simulink model "top_level_sim"  (R2024a)
settings: Solver=FixedStepAuto  StartTime=0.0  StopTime=10.0  FixedStep=0.01  RelTol=1e-3
InitFcn:
  | top_level_sim_init()
model workspace (MAT data in the model file):
  Kp_roll_regulator = 1
values from neighbouring files (symbols this model uses):
  cl03_as_kp = 0    [top_level_sim_init.m]
  cl03_climb_ki = 0    [top_level_sim_init.m]
  cl03_climb_kp = 0    [top_level_sim_init.m]
  cl03_pitch_ki = 0    [top_level_sim_init.m]
  cl03_pitch_kp = 0    [top_level_sim_init.m]
  cl03_roll_kp = 0    [top_level_sim_init.m]
  cl03_yaw_kp = 0    [top_level_sim_init.m]
  S_alphad0_ic_deg = rad2deg(atan2(S_wb0_ic_fps,S_ub0_ic_fps))    [top_level_sim_init.m]
  S_betad0_ic_deg = rad2deg(asin(S_vb0_ic_fps/norm([S_ub0_ic_fps,S_vb0_ic_fps, S_wb0_ic_fps])))    [top_level_sim_init.m]
  S_Ixx_ic_slf2 = 10^6    (= 1000000)    [top_level_sim_init.m]
  S_Ixy_ic_slf2 = 0    [top_level_sim_init.m]
  S_Iyy_ic_slf2 = 10^7    (= 10000000)    [top_level_sim_init.m]
  S_Iyz_ic_slf2 = 0    [top_level_sim_init.m]
  S_Izx_ic_slf2 = 0    [top_level_sim_init.m]
  S_Izz_ic_slf2 = 10^7    (= 10000000)    [top_level_sim_init.m]
  S_mass0_ic_lbs = 300000    [top_level_sim_init.m]
  S_pb0_ic_dps = rad2deg(S_pb0_ic_rps)    [top_level_sim_init.m]
  S_pb0_ic_rps = 0    [top_level_sim_init.m]
  S_phi0_ic_rad = 0    [top_level_sim_init.m]
  S_psi0_ic_rad = 0    [top_level_sim_init.m]
  S_qb0_ic_dps = rad2deg(S_qb0_ic_rps)    [top_level_sim_init.m]
  S_qb0_ic_rps = 0    [top_level_sim_init.m]
  S_rb0_ic_dps = rad2deg(S_rb0_ic_rps)    [top_level_sim_init.m]
  S_rb0_ic_rps = 0    [top_level_sim_init.m]
  S_theta0_ic_rad = 7    [top_level_sim_init.m]
  S_ub0_ic_fps = 5626    [top_level_sim_init.m]
  S_vb0_ic_fps = 0    [top_level_sim_init.m]
  S_wb0_ic_fps = 0    [top_level_sim_init.m]
  S_xi0_ic_ft = 0    [top_level_sim_init.m]
  S_yi0_ic_ft = 0    [top_level_sim_init.m]
  S_zi0_ic_ft = -200    [top_level_sim_init.m]
undefined symbols (not defined in the file or in its folder): CL04_Bmat0, DiscIntNeverNeededParam
libraries: simulink_extras x7, shared6dof x1, aerolibasang x1
settings Model: Creator=chrgutierrez  LastModifiedBy=chrgutierrez
settings DebuggingCC: UnconnectedInputMsg=warning  UnconnectedOutputMsg=warning  UnconnectedLineMsg=warning
settings ModelReferenceCC: EnableRefExpFcnMdlSchedulingChecks=on
settings RTWCC: GPUComputeCapability=3.5  DLArmComputeVersion=19.05

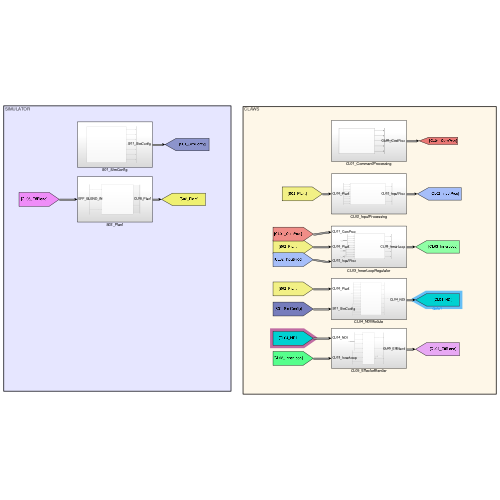
[thumbnail: Simulink's stored preview of the top-level diagram]
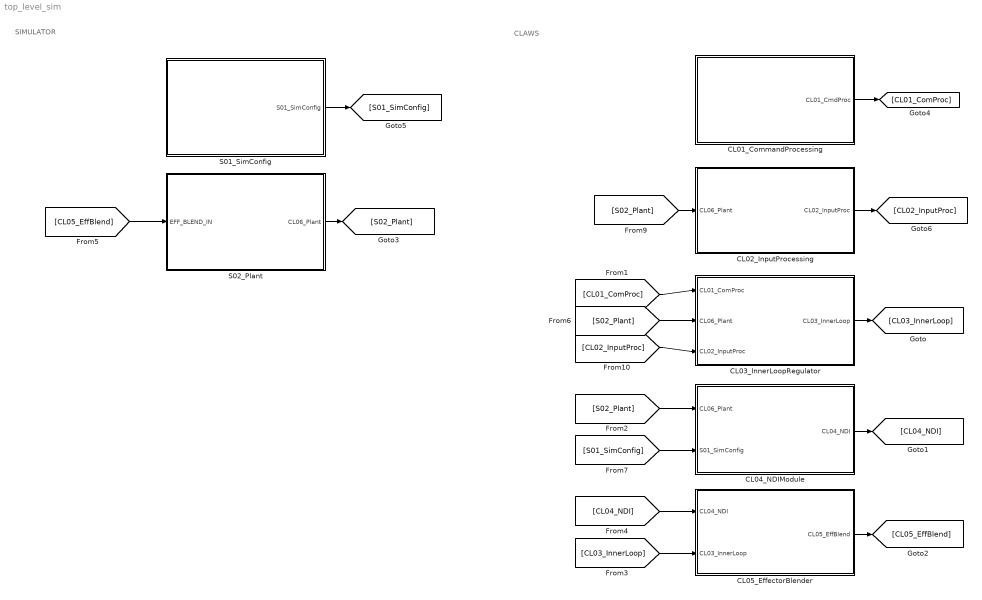
== system top_level_sim ==
  note: CLAWS
  note: SIMULATOR
  CL01_CommandProcessing : Subsystem
  CL02_InputProcessing : Subsystem
  CL03_InnerLoopRegulator : Subsystem
  CL04_NDIModule : Subsystem
  CL05_EffectorBlender : Subsystem
  S01_SimConfig : Subsystem
  S02_Plant : Subsystem
  wires:
  [S02_Plant] -> CL03_InnerLoopRegulator/2(CL06_Plant)
  [CL01_ComProc] -> CL03_InnerLoopRegulator/1(CL01_ComProc)
  CL03_InnerLoopRegulator/1(CL03_InnerLoop) -> [CL03_InnerLoop]
  [CL03_InnerLoop] -> CL05_EffectorBlender/2(CL03_InnerLoop)
  CL04_NDIModule/1(CL04_NDI) -> [CL04_NDI]
  [CL04_NDI] -> CL05_EffectorBlender/1(CL04_NDI)
  CL05_EffectorBlender/1(CL05_EffBlend) -> [CL05_EffBlend]
  [CL05_EffBlend] -> S02_Plant/1(EFF_BLEND_IN)
  [S02_Plant] -> CL04_NDIModule/1(CL06_Plant)
  S01_SimConfig/1(S01_SimConfig) -> [S01_SimConfig]
  [S01_SimConfig] -> CL04_NDIModule/2(S01_SimConfig)
  [S02_Plant] -> CL02_InputProcessing/1(CL06_Plant)
  CL02_InputProcessing/1(CL02_InputProc) -> [CL02_InputProc]
  S02_Plant/1(CL06_Plant) -> [S02_Plant]
  [CL02_InputProc] -> CL03_InnerLoopRegulator/3(CL02_InputProc)
  CL01_CommandProcessing/1(CL01_CmdProc) -> [CL01_ComProc]

== system top_level_sim/CL01_CommandProcessing ==
  Bus Creator : BusCreator  Inputs=5  OutDataTypeStr=Bus: B_CL01_ComProc
      settings: InheritFromInputs=off
  Subsystem : Subsystem
  CL01_CmdProc : Outport
  wires:
  Subsystem/3(rb_cmd_dps) -> Bus Creator/3
  Subsystem/2(qb_cmd_dps) -> Bus Creator/2
  Subsystem/1(pb_cmd_dps) -> Bus Creator/1
  Subsystem/4(as_cmd_fps) -> Bus Creator/4
  Subsystem/5(climb_cmd_fps) -> Bus Creator/5
  Bus Creator/1 -> CL01_CmdProc/1

== system top_level_sim/CL02_InputProcessing ==
  CL06_Plant : Inport
  Bus Creator : BusCreator  Inputs=3  OutDataTypeStr=Bus: B_CL02_InputProcessing
      settings: InheritFromInputs=off
  Bus Selector : BusSelector  OutputSignals=phi_state_rad,theta_state_rad,psi_state_rad,vnorth_state_fps,veast_state_fps,vup_state_fps,ub_state_fps,vb_state_fps,wb_state_fps
  Subsystem : Subsystem
  CL02_InputProc : Outport
  wires:
  CL06_Plant/1 -> Bus Selector/1
  Bus Selector/9 -> Subsystem/9(wb_state_fps)  "<wb_state_fps>"
  Bus Selector/8 -> Subsystem/8(vb_state_fps)  "<vb_state_fps>"
  Bus Selector/7 -> Subsystem/7(ub_state_fps)  "<ub_state_fps>"
  Bus Selector/6 -> Subsystem/6(vup_state_fps)  "<vup_state_fps>"
  Bus Selector/5 -> Subsystem/5(veast_state_fps)  "<veast_state_fps>"
  Bus Selector/4 -> Subsystem/4(vnorth_state_fps)  "<vnorth_state_fps>"
  Bus Selector/3 -> Subsystem/3(psi_state_rad)  "<psi_state_rad>"
  Bus Selector/2 -> Subsystem/2(theta_state_rad)  "<theta_state_rad>"
  Bus Selector/1 -> Subsystem/1(phi_state_rad)  "<phi_state_rad>"
  Subsystem/3(aoa_i_proc_deg) -> Bus Creator/3
  Subsystem/2(aos_i_proc_deg) -> Bus Creator/2
  Subsystem/1(vtot_i_proc_fps) -> Bus Creator/1
  Bus Creator/1 -> CL02_InputProc/1

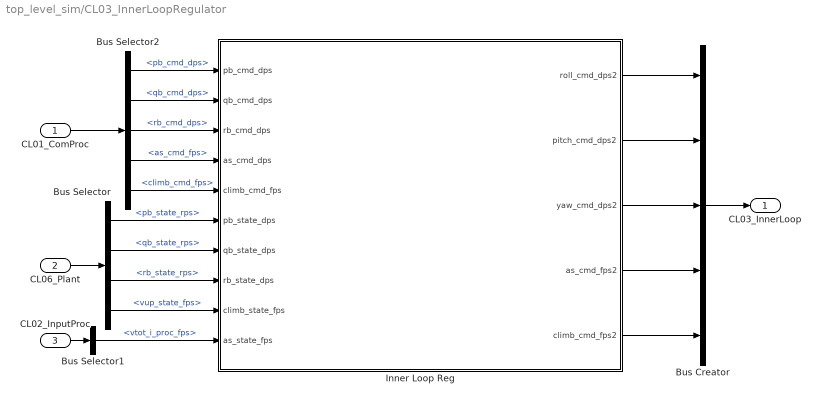
== system top_level_sim/CL03_InnerLoopRegulator ==
  CL01_ComProc : Inport
  CL06_Plant : Inport  Port=2
  CL02_InputProc : Inport  Port=3
  Bus Creator : BusCreator  Inputs=5  OutDataTypeStr=Bus: B_CL03_InnerLoop
      settings: InheritFromInputs=off
  Bus Selector : BusSelector  OutputSignals=pb_state_rps,qb_state_rps,rb_state_rps,vup_state_fps
  Bus Selector1 : BusSelector  OutputSignals=vtot_i_proc_fps
  Bus Selector2 : BusSelector  OutputSignals=pb_cmd_dps,qb_cmd_dps,rb_cmd_dps,as_cmd_fps,climb_cmd_fps
  Inner Loop Reg : Subsystem
  CL03_InnerLoop : Outport
  wires:
  Inner Loop Reg/5(climb_cmd_fps2) -> Bus Creator/5
  Inner Loop Reg/1(roll_cmd_dps2) -> Bus Creator/1
  Inner Loop Reg/4(as_cmd_fps2) -> Bus Creator/4
  Inner Loop Reg/3(yaw_cmd_dps2) -> Bus Creator/3
  Inner Loop Reg/2(pitch_cmd_dps2) -> Bus Creator/2
  Bus Creator/1 -> CL03_InnerLoop/1
  CL06_Plant/1 -> Bus Selector/1
  Bus Selector/1 -> Inner Loop Reg/6(pb_state_dps)  "<pb_state_rps>"
  Bus Selector/2 -> Inner Loop Reg/7(qb_state_dps)  "<qb_state_rps>"
  Bus Selector/3 -> Inner Loop Reg/8(rb_state_dps)  "<rb_state_rps>"
  Bus Selector/4 -> Inner Loop Reg/9(climb_state_fps)  "<vup_state_fps>"
  CL02_InputProc/1 -> Bus Selector1/1
  Bus Selector1/1 -> Inner Loop Reg/10(as_state_fps)  "<vtot_i_proc_fps>"
  CL01_ComProc/1 -> Bus Selector2/1
  Bus Selector2/1 -> Inner Loop Reg/1(pb_cmd_dps)  "<pb_cmd_dps>"
  Bus Selector2/2 -> Inner Loop Reg/2(qb_cmd_dps)  "<qb_cmd_dps>"
  Bus Selector2/3 -> Inner Loop Reg/3(rb_cmd_dps)  "<rb_cmd_dps>"
  Bus Selector2/4 -> Inner Loop Reg/4(as_cmd_dps)  "<as_cmd_fps>"
  Bus Selector2/5 -> Inner Loop Reg/5(climb_cmd_fps)  "<climb_cmd_fps>"

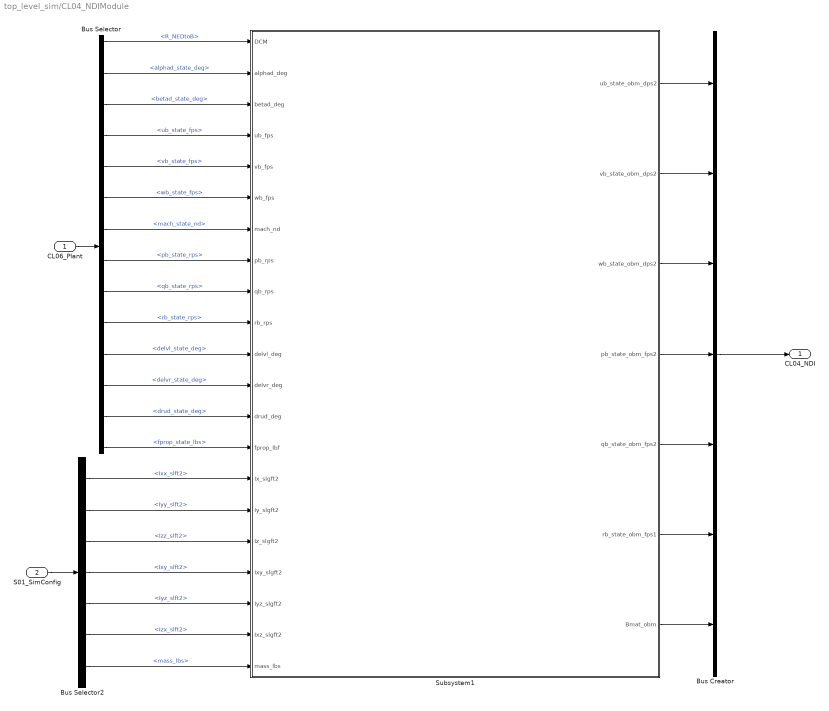
== system top_level_sim/CL04_NDIModule ==
  CL06_Plant : Inport
  S01_SimConfig : Inport  Port=2
  Bus Creator : BusCreator  Inputs=7  OutDataTypeStr=Bus: B_CL04_NDI
      settings: InheritFromInputs=off
  Bus Selector : BusSelector  OutputSignals=R_NEDtoB,alphad_state_deg,betad_state_deg,ub_state_fps,vb_state_fps,wb_state_fps,mach_state_nd,pb_state_rps,qb_state_rps,rb_state_rps,delvl_state_deg,delvr_state_deg,drud_state_deg,fprop_state_lbs
  Bus Selector2 : BusSelector  OutputSignals=Ixx_slft2,Iyy_slft2,Izz_slft2,Ixy_slft2,Iyz_slft2,Izx_slft2,mass_lbs
  Subsystem1 : Subsystem
  CL04_NDI : Outport
  wires:
  CL06_Plant/1 -> Bus Selector/1
  Subsystem1/4(pb_state_obm_fps2) -> Bus Creator/4
  Subsystem1/3(wb_state_obm_dps2) -> Bus Creator/3
  Subsystem1/2(vb_state_obm_dps2) -> Bus Creator/2
  Subsystem1/1(ub_state_obm_dps2) -> Bus Creator/1
  Bus Creator/1 -> CL04_NDI/1
  S01_SimConfig/1 -> Bus Selector2/1
  Bus Selector2/7 -> Subsystem1/21(mass_lbs)  "<mass_lbs>"
  Bus Selector2/1 -> Subsystem1/15(Ix_slgft2)  "<Ixx_slft2>"
  Bus Selector2/2 -> Subsystem1/16(Iy_slgft2)  "<Iyy_slft2>"
  Bus Selector2/3 -> Subsystem1/17(Iz_slgft2)  "<Izz_slft2>"
  Bus Selector2/6 -> Subsystem1/20(Ixz_slgft2)  "<Izx_slft2>"
  Bus Selector2/5 -> Subsystem1/19(Iyz_slgft2)  "<Iyz_slft2>"
  Bus Selector2/4 -> Subsystem1/18(Ixy_slgft2)  "<Ixy_slft2>"
  Bus Selector/2 -> Subsystem1/2(alphad_deg)  "<alphad_state_deg>"
  Bus Selector/3 -> Subsystem1/3(betad_deg)  "<betad_state_deg>"
  Bus Selector/4 -> Subsystem1/4(ub_fps)  "<ub_state_fps>"
  Bus Selector/5 -> Subsystem1/5(vb_fps)  "<vb_state_fps>"
  Bus Selector/6 -> Subsystem1/6(wb_fps)  "<wb_state_fps>"
  Bus Selector/8 -> Subsystem1/8(pb_rps)  "<pb_state_rps>"
  Bus Selector/9 -> Subsystem1/9(qb_rps)  "<qb_state_rps>"
  Bus Selector/10 -> Subsystem1/10(rb_rps)  "<rb_state_rps>"
  Subsystem1/5(qb_state_obm_fps2) -> Bus Creator/5
  Bus Selector/11 -> Subsystem1/11(delvl_deg)  "<delvl_state_deg>"
  Bus Selector/12 -> Subsystem1/12(delvr_deg)  "<delvr_state_deg>"
  Bus Selector/13 -> Subsystem1/13(drud_deg)  "<drud_state_deg>"
  Bus Selector/14 -> Subsystem1/14(fprop_lbf)  "<fprop_state_lbs>"
  Bus Selector/1 -> Subsystem1/1(DCM)  "<R_NEDtoB>"
  Bus Selector/7 -> Subsystem1/7(mach_nd)  "<mach_state_nd>"
  Subsystem1/7(Bmat_obm) -> Bus Creator/7
  Subsystem1/6(rb_state_obm_fps1) -> Bus Creator/6

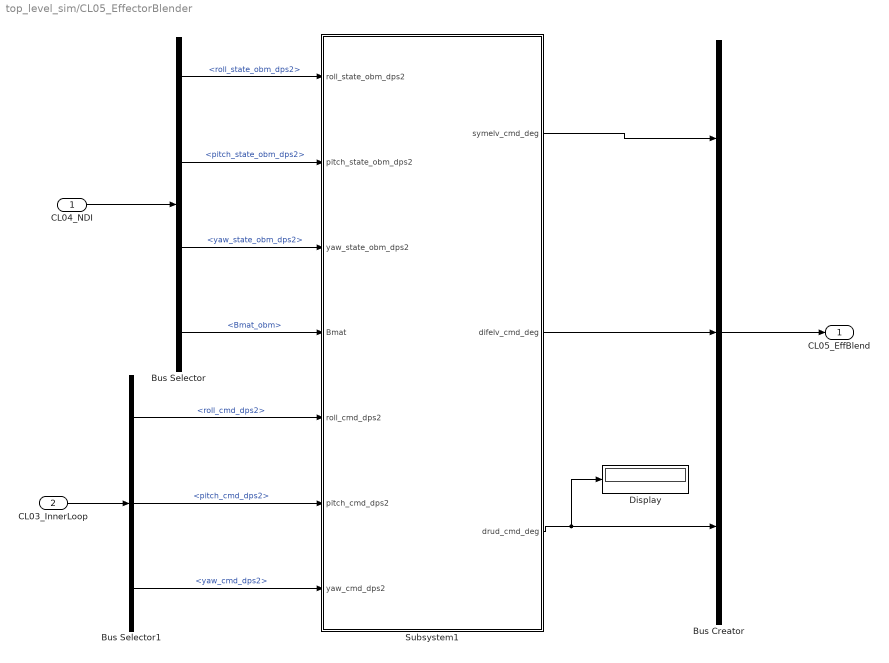
== system top_level_sim/CL05_EffectorBlender ==
  CL04_NDI : Inport
  CL03_InnerLoop : Inport  Port=2
  Bus Creator : BusCreator  Inputs=3  OutDataTypeStr=Bus: B_CL05_EffBlend
      settings: InheritFromInputs=off
  Bus Selector : BusSelector  OutputSignals=roll_state_obm_dps2,pitch_state_obm_dps2,yaw_state_obm_dps2,Bmat_obm
  Bus Selector1 : BusSelector  OutputSignals=roll_cmd_dps2,pitch_cmd_dps2,yaw_cmd_dps2
  Display : Display
  Subsystem1 : Subsystem
  CL05_EffBlend : Outport
  wires:
  CL04_NDI/1 -> Bus Selector/1
  CL03_InnerLoop/1 -> Bus Selector1/1
  Subsystem1/1(symelv_cmd_deg) -> Bus Creator/1
  Subsystem1/2(difelv_cmd_deg) -> Bus Creator/2
  Subsystem1/3(drud_cmd_deg) -> Display/1, Bus Creator/3
  Bus Creator/1 -> CL05_EffBlend/1
  Bus Selector/1 -> Subsystem1/1(roll_state_obm_dps2)  "<roll_state_obm_dps2>"
  Bus Selector/2 -> Subsystem1/2(pitch_state_obm_dps2)  "<pitch_state_obm_dps2>"
  Bus Selector/3 -> Subsystem1/3(yaw_state_obm_dps2)  "<yaw_state_obm_dps2>"
  Bus Selector/4 -> Subsystem1/4(Bmat)  "<Bmat_obm>"
  Bus Selector1/3 -> Subsystem1/7(yaw_cmd_dps2)  "<yaw_cmd_dps2>"
  Bus Selector1/2 -> Subsystem1/6(pitch_cmd_dps2)  "<pitch_cmd_dps2>"
  Bus Selector1/1 -> Subsystem1/5(roll_cmd_dps2)  "<roll_cmd_dps2>"

== system top_level_sim/S01_SimConfig ==
  Bus Creator : BusCreator  Inputs=7  OutDataTypeStr=Bus: B_S01_SimConfig
      settings: InheritFromInputs=off
  Subsystem : Subsystem
  S01_SimConfig : Outport
  wires:
  Bus Creator/1 -> S01_SimConfig/1
  Subsystem/1(mass_lbs) -> Bus Creator/1
  Subsystem/2(Ixx_slft2) -> Bus Creator/2
  Subsystem/3(Iyy_slft2) -> Bus Creator/3
  Subsystem/4(Izz_slft2) -> Bus Creator/4
  Subsystem/5(Ixy_slft2) -> Bus Creator/5
  Subsystem/6(Iyz_slft2) -> Bus Creator/6
  Subsystem/7(Izx_slft2) -> Bus Creator/7

== system top_level_sim/S02_Plant ==
  EFF_BLEND_IN : Inport
  Bus Creator : BusCreator  Inputs=29  OutDataTypeStr=Bus: B_S02_Plant
      settings: InheritFromInputs=off
  Bus Selector : BusSelector  OutputSignals=symelv_cmd_deg,difelv_cmd_deg,drud_cmd_deg
  Subsystem : Subsystem
  CL06_Plant : Outport
  wires:
  Bus Creator/1 -> CL06_Plant/1
  EFF_BLEND_IN/1 -> Bus Selector/1
  Subsystem/1(alphad_deg1) -> Bus Creator/1
  Subsystem/2(betad_deg1) -> Bus Creator/2
  Subsystem/3(delvl_state_deg) -> Bus Creator/3
  Subsystem/4(delvr_state_deg) -> Bus Creator/4
  Subsystem/5(drud_state_deg) -> Bus Creator/5
  Subsystem/6(fprop_state_lbf) -> Bus Creator/6
  Subsystem/7(vnorth_state_fps) -> Bus Creator/7
  Subsystem/8(veast_state_fps) -> Bus Creator/8
  Subsystem/9(vup_state_fps) -> Bus Creator/9
  Subsystem/10(xnorth_state_ft) -> Bus Creator/10
  Subsystem/11(xeast_state_ft) -> Bus Creator/11
  Subsystem/12(xup_state_ft) -> Bus Creator/12
  Subsystem/13(phi_state_rad) -> Bus Creator/13
  Subsystem/14(theta_state_rad) -> Bus Creator/14
  Subsystem/15(psi_state_rad) -> Bus Creator/15
  Subsystem/16(R_NEDtoB) -> Bus Creator/16
  Subsystem/17(ub_state_fps) -> Bus Creator/17
  Subsystem/18(vb_state_fps) -> Bus Creator/18
  Subsystem/19(wb_state_fps) -> Bus Creator/19
  Subsystem/20(pb_state_rps) -> Bus Creator/20
  Subsystem/21(qb_state_rps) -> Bus Creator/21
  Subsystem/22(rb_state_rps) -> Bus Creator/22
  Subsystem/23(pbdot_state_rps2) -> Bus Creator/23
  Subsystem/24(qbdot_state_rps2) -> Bus Creator/24
  Subsystem/25(rbdot_state_rps2) -> Bus Creator/25
  Subsystem/26(axb_state_fps2) -> Bus Creator/26
  Subsystem/27(ayb_state_fps2) -> Bus Creator/27
  Subsystem/28(azb_state_fps2) -> Bus Creator/28
  Bus Selector/2 -> Subsystem/2(difelv_cmd_deg)  "<difelv_cmd_deg>"
  Bus Selector/1 -> Subsystem/1(symelv_cmd_deg)  "<symelv_cmd_deg>"
  Bus Selector/3 -> Subsystem/3(drud_deg)  "<drud_cmd_deg>"
  Subsystem/29(mach_state_nd) -> Bus Creator/29

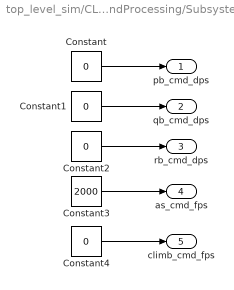
== system top_level_sim/CL01_CommandProcessing/Subsystem ==
  Constant{,1..2,4} (4 alike) : Constant  Value=0
  Constant3 : Constant  Value=2000
  pb_cmd_dps : Outport
  qb_cmd_dps : Outport  Port=2
  rb_cmd_dps : Outport  Port=3
  as_cmd_fps : Outport  Port=4
  climb_cmd_fps : Outport  Port=5
  wires:
  Constant/1 -> pb_cmd_dps/1
  Constant1/1 -> qb_cmd_dps/1
  Constant2/1 -> rb_cmd_dps/1
  Constant3/1 -> as_cmd_fps/1
  Constant4/1 -> climb_cmd_fps/1

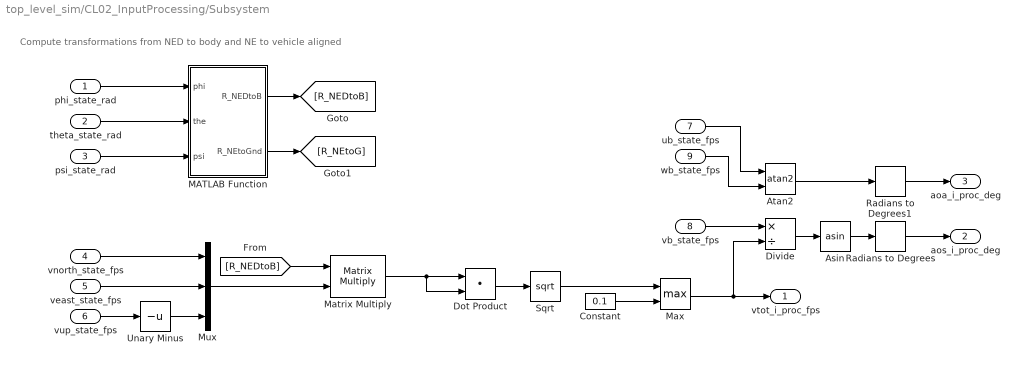
== system top_level_sim/CL02_InputProcessing/Subsystem ==
  note: Compute transformations from NED to body and NE to vehicle aligned
  phi_state_rad : Inport
  theta_state_rad : Inport  Port=2
  psi_state_rad : Inport  Port=3
  vnorth_state_fps : Inport  Port=4
  veast_state_fps : Inport  Port=5
  vup_state_fps : Inport  Port=6
  ub_state_fps : Inport  Port=7
  vb_state_fps : Inport  Port=8
  wb_state_fps : Inport  Port=9
  Asin : Trigonometry  Operator=asin
  Atan2 : Trigonometry  Operator=atan2
  Constant : Constant  Value=0.1
  Divide : Product  Inputs=*/
  Dot Product : DotProduct  OutDataTypeStr=Inherit: Inherit via internal rule
  MATLAB Function : MATLAB Function  TreatAsAtomicUnit=on
  Matrix Multiply : Product  Multiplication=Matrix(*)
  Max : MinMax  Function=max  Inputs=2
  Mux : Mux  Inputs=3
  Radians to Degrees : simulink_extras/Transformations/Radians to Degrees
  Radians to Degrees1 : simulink_extras/Transformations/Radians to Degrees
  Sqrt : Sqrt
  Unary Minus : UnaryMinus
  vtot_i_proc_fps : Outport
  aos_i_proc_deg : Outport  Port=2
  aoa_i_proc_deg : Outport  Port=3
  wires:
  psi_state_rad/1 -> MATLAB Function/3(psi)
  theta_state_rad/1 -> MATLAB Function/2(the)
  phi_state_rad/1 -> MATLAB Function/1(phi)
  MATLAB Function/2(R_NEtoGnd) -> [R_NEtoG]
  MATLAB Function/1(R_NEDtoB) -> [R_NEDtoB]
  vup_state_fps/1 -> Unary Minus/1
  veast_state_fps/1 -> Mux/2
  vnorth_state_fps/1 -> Mux/1
  Unary Minus/1 -> Mux/3
  Mux/1 -> Matrix Multiply/2
  [R_NEDtoB] -> Matrix Multiply/1
  Matrix Multiply/1 -> Dot Product/1, Dot Product/2
  Dot Product/1 -> Sqrt/1
  Sqrt/1 -> Max/1
  Constant/1 -> Max/2
  Max/1 -> vtot_i_proc_fps/1, Divide/2
  vb_state_fps/1 -> Divide/1
  Divide/1 -> Asin/1
  Asin/1 -> Radians to Degrees/1
  Radians to Degrees/1 -> aos_i_proc_deg/1
  wb_state_fps/1 -> Atan2/2
  ub_state_fps/1 -> Atan2/1
  Atan2/1 -> Radians to Degrees1/1
  Radians to Degrees1/1 -> aoa_i_proc_deg/1

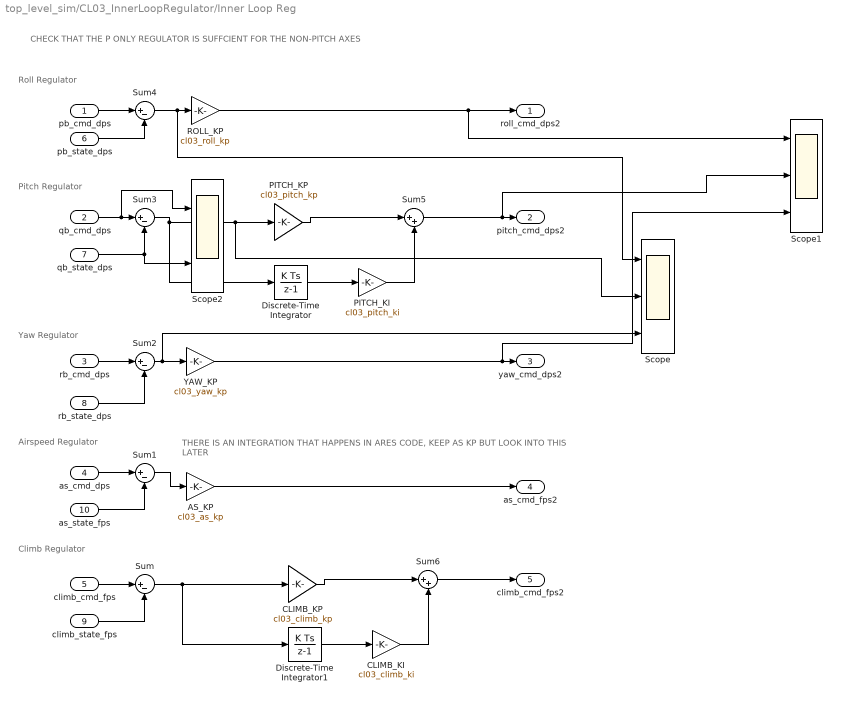
== system top_level_sim/CL03_InnerLoopRegulator/Inner Loop Reg ==
  note: THERE IS AN INTEGRATION THAT HAPPENS IN ARES CODE, KEEP AS KP BUT LOOK INTO THIS LATER
  note: CHECK THAT THE P ONLY REGULATOR IS SUFFCIENT FOR THE NON-PITCH AXES
  note: Roll Regulator
  note: Pitch Regulator
  note: Yaw Regulator
  note: Airspeed Regulator
  note: Climb Regulator
  pb_cmd_dps : Inport
  qb_cmd_dps : Inport  Port=2
  rb_cmd_dps : Inport  Port=3
  as_cmd_dps : Inport  Port=4
  climb_cmd_fps : Inport  Port=5
  pb_state_dps : Inport  Port=6
  qb_state_dps : Inport  Port=7
  rb_state_dps : Inport  Port=8
  climb_state_fps : Inport  Port=9
  as_state_fps : Inport  Port=10
  AS_KP : Gain  Gain=cl03_as_kp
  CLIMB_KI : Gain  Gain=cl03_climb_ki
  CLIMB_KP : Gain  Gain=cl03_climb_kp
  Discrete-Time Integrator : DiscreteIntegrator  SampleTime=-1  ICPrevOutput=DiscIntNeverNeededParam  ICPrevScaledInput=DiscIntNeverNeededParam
  Discrete-Time Integrator1 : DiscreteIntegrator  SampleTime=-1  ICPrevOutput=DiscIntNeverNeededParam  ICPrevScaledInput=DiscIntNeverNeededParam
  PITCH_KI : Gain  Gain=cl03_pitch_ki
  PITCH_KP : Gain  Gain=cl03_pitch_kp
  ROLL_KP : Gain  Gain=cl03_roll_kp
  Scope : Scope  NumInputPorts=3
  Scope1 : Scope  NumInputPorts=3
  Scope2 : Scope  NumInputPorts=2
  Sum{,1..4} (5 alike) : Sum  Inputs=|+-
  Sum5 : Sum  Inputs=|++
  Sum6 : Sum  Inputs=|++
  YAW_KP : Gain  Gain=cl03_yaw_kp
  roll_cmd_dps2 : Outport
  pitch_cmd_dps2 : Outport  Port=2
  yaw_cmd_dps2 : Outport  Port=3
  as_cmd_fps2 : Outport  Port=4
  climb_cmd_fps2 : Outport  Port=5
  wires:
  climb_cmd_fps/1 -> Sum/1
  climb_state_fps/1 -> Sum/2
  as_cmd_dps/1 -> Sum1/1
  as_state_fps/1 -> Sum1/2
  rb_cmd_dps/1 -> Sum2/1
  rb_state_dps/1 -> Sum2/2
  qb_cmd_dps/1 -> Scope2/1, Sum3/1
  qb_state_dps/1 -> Scope2/2, Sum3/2
  pb_cmd_dps/1 -> Sum4/1
  pb_state_dps/1 -> Sum4/2
  Sum4/1 -> Scope/1, ROLL_KP/1
  ROLL_KP/1 -> Scope1/1, roll_cmd_dps2/1
  Sum2/1 -> Scope/3, YAW_KP/1
  YAW_KP/1 -> Scope1/3, yaw_cmd_dps2/1
  Sum1/1 -> AS_KP/1
  AS_KP/1 -> as_cmd_fps2/1
  Discrete-Time Integrator/1 -> PITCH_KI/1
  PITCH_KI/1 -> Sum5/2
  PITCH_KP/1 -> Sum5/1
  Sum5/1 -> Scope1/2, pitch_cmd_dps2/1
  Sum3/1 -> Scope/2, PITCH_KP/1, Discrete-Time Integrator/1
  Sum/1 -> CLIMB_KP/1, Discrete-Time Integrator1/1
  Sum6/1 -> climb_cmd_fps2/1
  CLIMB_KI/1 -> Sum6/2
  Discrete-Time Integrator1/1 -> CLIMB_KI/1
  CLIMB_KP/1 -> Sum6/1

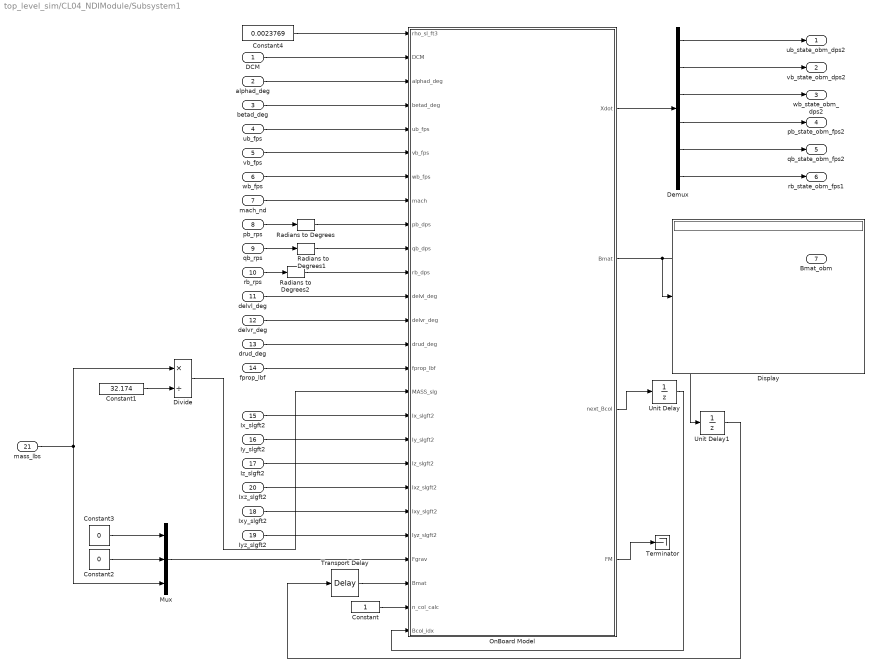
== system top_level_sim/CL04_NDIModule/Subsystem1 ==
  DCM : Inport
  alphad_deg : Inport  Port=2
  betad_deg : Inport  Port=3
  ub_fps : Inport  Port=4
  vb_fps : Inport  Port=5
  wb_fps : Inport  Port=6
  mach_nd : Inport  Port=7
  pb_rps : Inport  Port=8
  qb_rps : Inport  Port=9
  rb_rps : Inport  Port=10
  delvl_deg : Inport  Port=11
  delvr_deg : Inport  Port=12
  drud_deg : Inport  Port=13
  fprop_lbf : Inport  Port=14
  Ix_slgft2 : Inport  Port=15
  Iy_slgft2 : Inport  Port=16
  Iz_slgft2 : Inport  Port=17
  Ixy_slgft2 : Inport  Port=18
  Iyz_slgft2 : Inport  Port=19
  Ixz_slgft2 : Inport  Port=20
  mass_lbs : Inport  Port=21
  Constant : Constant
  Constant1 : Constant  Value=32.174
  Constant2 : Constant  Value=0
  Constant3 : Constant  Value=0
  Constant4 : Constant  Value=0.0023769
  Demux : Demux  Outputs=6
  Display : Display
  Divide : Product  Inputs=*/
  Mux : Mux  Inputs=3
  OnBoard Model : MATLAB Function  TreatAsAtomicUnit=on
  Radians to Degrees : simulink_extras/Transformations/Radians to Degrees
  Radians to Degrees1 : simulink_extras/Transformations/Radians to Degrees
  Radians to Degrees2 : simulink_extras/Transformations/Radians to Degrees
  Terminator : Terminator
  Transport Delay : TransportDelay  DelayTime=3  InitialOutput=CL04_Bmat0
  Unit Delay : UnitDelay  SampleTime=-1  HasFrameUpgradeWarning=on
  Unit Delay1 : UnitDelay  SampleTime=-1  HasFrameUpgradeWarning=on
  ub_state_obm_dps2 : Outport
  vb_state_obm_dps2 : Outport  Port=2
  wb_state_obm_dps2 : Outport  Port=3
  pb_state_obm_fps2 : Outport  Port=4
  qb_state_obm_fps2 : Outport  Port=5
  rb_state_obm_fps1 : Outport  Port=6
  Bmat_obm : Outport  Port=7
  wires:
  OnBoard Model/3(next_Bcol) -> Unit Delay/1
  OnBoard Model/2(Bmat) -> Display/1, Unit Delay1/1, Bmat_obm/1
  OnBoard Model/4(FM) -> Terminator/1
  OnBoard Model/1(Xdot) -> Demux/1
  Unit Delay/1 -> OnBoard Model/26(Bcol_idx)
  Demux/3 -> wb_state_obm_dps2/1
  Demux/1 -> ub_state_obm_dps2/1
  Demux/2 -> vb_state_obm_dps2/1
  Demux/4 -> pb_state_obm_fps2/1
  Demux/5 -> qb_state_obm_fps2/1
  Unit Delay1/1 -> Transport Delay/1
  Constant/1 -> OnBoard Model/25(n_col_calc)
  wb_fps/1 -> OnBoard Model/7(wb_fps)
  vb_fps/1 -> OnBoard Model/6(vb_fps)
  ub_fps/1 -> OnBoard Model/5(ub_fps)
  Ix_slgft2/1 -> OnBoard Model/17(Ix_slgft2)
  Iy_slgft2/1 -> OnBoard Model/18(Iy_slgft2)
  Iz_slgft2/1 -> OnBoard Model/19(Iz_slgft2)
  Ixz_slgft2/1 -> OnBoard Model/20(Ixz_slgft2)
  Ixy_slgft2/1 -> OnBoard Model/21(Ixy_slgft2)
  Iyz_slgft2/1 -> OnBoard Model/22(Iyz_slgft2)
  delvl_deg/1 -> OnBoard Model/12(delvl_deg)
  drud_deg/1 -> OnBoard Model/14(drud_deg)
  delvr_deg/1 -> OnBoard Model/13(delvr_deg)
  pb_rps/1 -> Radians to Degrees/1
  Radians to Degrees/1 -> OnBoard Model/9(pb_dps)
  qb_rps/1 -> Radians to Degrees1/1
  Radians to Degrees1/1 -> OnBoard Model/10(qb_dps)
  rb_rps/1 -> Radians to Degrees2/1
  Radians to Degrees2/1 -> OnBoard Model/11(rb_dps)
  alphad_deg/1 -> OnBoard Model/3(alphad_deg)
  betad_deg/1 -> OnBoard Model/4(betad_deg)
  Constant1/1 -> Divide/2
  mass_lbs/1 -> Divide/1, Mux/3
  Divide/1 -> OnBoard Model/16(MASS_slg)
  fprop_lbf/1 -> OnBoard Model/15(fprop_lbf)
  Constant3/1 -> Mux/1
  Constant2/1 -> Mux/2
  Mux/1 -> OnBoard Model/23(Fgrav)
  DCM/1 -> OnBoard Model/2(DCM)
  Constant4/1 -> OnBoard Model/1(rho_sl_ft3)
  mach_nd/1 -> OnBoard Model/8(mach)
  Demux/6 -> rb_state_obm_fps1/1
  Transport Delay/1 -> OnBoard Model/24("Bmat ")

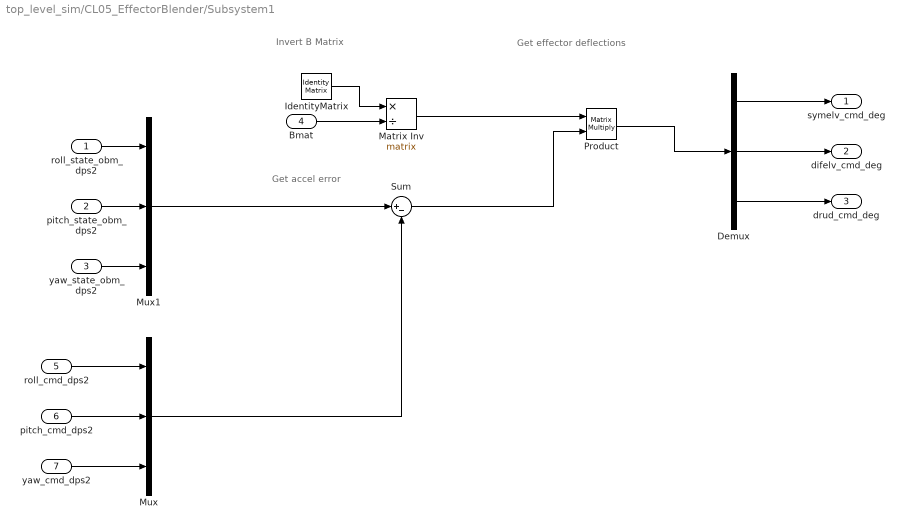
== system top_level_sim/CL05_EffectorBlender/Subsystem1 ==
  note: Get accel error
  note: Invert B Matrix
  note: Get effector deflections
  roll_state_obm_dps2 : Inport
  pitch_state_obm_dps2 : Inport  Port=2
  yaw_state_obm_dps2 : Inport  Port=3
  Bmat : Inport  Port=4
  roll_cmd_dps2 : Inport  Port=5
  pitch_cmd_dps2 : Inport  Port=6
  yaw_cmd_dps2 : Inport  Port=7
  Demux : Demux  Outputs=3
  IdentityMatrix : IdentityMatrix  OutputDimensions=3
  Matrix Inv : Product  Inputs=*/  Multiplication=Matrix(*)
  Mux : Mux  Inputs=3
  Mux1 : Mux  Inputs=3
  Product : Product  Multiplication=Matrix(*)
  Sum : Sum  Inputs=|+-
  symelv_cmd_deg : Outport
  difelv_cmd_deg : Outport  Port=2
  drud_cmd_deg : Outport  Port=3
  wires:
  Matrix Inv/1 -> Product/1
  Sum/1 -> Product/2
  Bmat/1 -> Matrix Inv/2
  IdentityMatrix/1 -> Matrix Inv/1
  Demux/2 -> difelv_cmd_deg/1
  Demux/3 -> drud_cmd_deg/1
  Demux/1 -> symelv_cmd_deg/1
  Product/1 -> Demux/1
  yaw_state_obm_dps2/1 -> Mux1/3
  pitch_state_obm_dps2/1 -> Mux1/2
  roll_state_obm_dps2/1 -> Mux1/1
  Mux1/1 -> Sum/1
  yaw_cmd_dps2/1 -> Mux/3
  pitch_cmd_dps2/1 -> Mux/2
  roll_cmd_dps2/1 -> Mux/1
  Mux/1 -> Sum/2

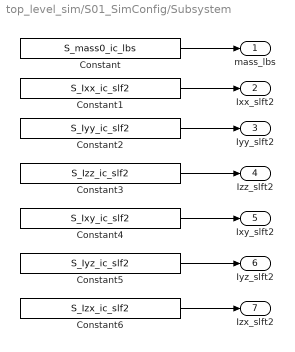
== system top_level_sim/S01_SimConfig/Subsystem ==
  Constant : Constant  Value=S_mass0_ic_lbs
  Constant1 : Constant  Value=S_Ixx_ic_slf2
  Constant2 : Constant  Value=S_Iyy_ic_slf2
  Constant3 : Constant  Value=S_Izz_ic_slf2
  Constant4 : Constant  Value=S_Ixy_ic_slf2
  Constant5 : Constant  Value=S_Iyz_ic_slf2
  Constant6 : Constant  Value=S_Izx_ic_slf2
  mass_lbs : Outport
  Ixx_slft2 : Outport  Port=2
  Iyy_slft2 : Outport  Port=3
  Izz_slft2 : Outport  Port=4
  Ixy_slft2 : Outport  Port=5
  Iyz_slft2 : Outport  Port=6
  Izx_slft2 : Outport  Port=7
  wires:
  Constant/1 -> mass_lbs/1
  Constant1/1 -> Ixx_slft2/1
  Constant2/1 -> Iyy_slft2/1
  Constant3/1 -> Izz_slft2/1
  Constant6/1 -> Izx_slft2/1
  Constant5/1 -> Iyz_slft2/1
  Constant4/1 -> Ixy_slft2/1

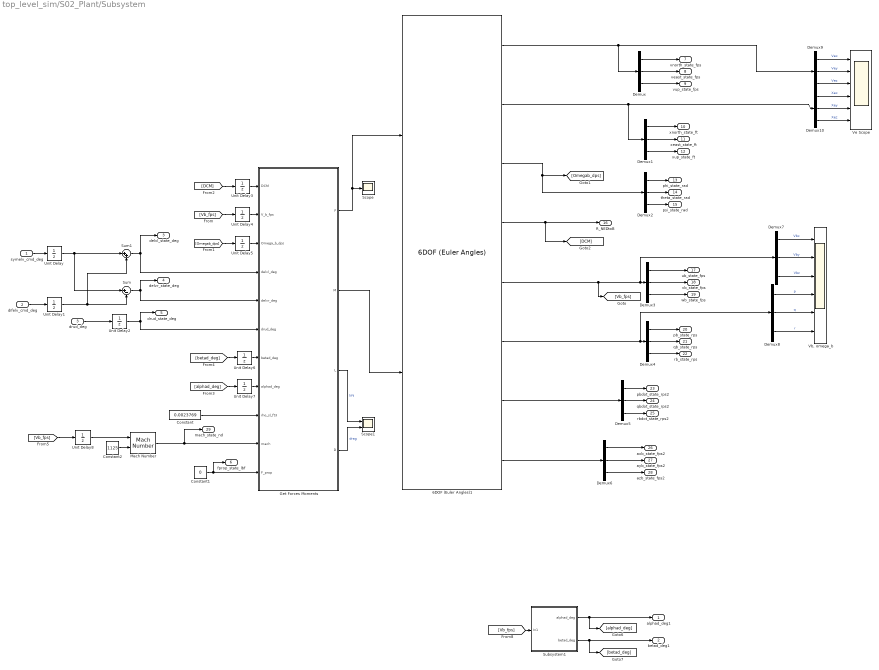
== system top_level_sim/S02_Plant/Subsystem ==
  symelv_cmd_deg : Inport
  difelv_cmd_deg : Inport  Port=2
  drud_deg : Inport  Port=3
  6DOF (Euler Angles)1 : shared6dof/6DOF (Euler Angles)  units=English (Velocity in ft/s)  mtype=Fixed  rep=Euler Angles  xme_0=[S_xi0_ic_ft S_yi0_ic_ft S_zi0_ic_ft]  Vm_0=[S_ub0_ic_fps, S_vb0_ic_fps, S_wb0_ic_fps]  eul_0=[S_phi0_ic_rad, S_theta0_ic_rad, S_psi0_ic_rad]  pm_0=[S_pb0_ic_rps S_qb0_ic_rps S_rb0_ic_rps]  mass_0=S_mass0_ic_lbs  mass_e=0.5  mass_f=2.0  inertia=diag([S_Ixx_ic_slf2,S_Iyy_ic_slf2,S_Izz_ic_slf2])  inertia_e=eye(3)  inertia_f=2*eye(3)  k_quat=1.0  vre_flag=on  abi_flag=off  aMode=0  xme_statename=''  Vm_statename=''  eul_statename=''  quat_statename=''  pm_statename=''  mass_statename=''
  Constant : Constant  Value=0.0023769
  Constant1 : Constant  Value=0
  Constant2 : Constant  Value=1125
  Demux{,1..10} (11 alike) : Demux  Outputs=3
  Get Forces Moments : MATLAB Function  TreatAsAtomicUnit=on
  Mach Number : aerolibasang/Mach Number
  Scope : Scope
  Scope1 : Scope  NumInputPorts=2
  Subsystem1 : Subsystem
  Sum : Sum  Inputs=|+-
  Sum1 : Sum  Inputs=|++
  Unit Delay : UnitDelay  SampleTime=-1  HasFrameUpgradeWarning=on
  Unit Delay1 : UnitDelay  SampleTime=-1  HasFrameUpgradeWarning=on
  Unit Delay2 : UnitDelay  SampleTime=-1  HasFrameUpgradeWarning=on
  Unit Delay3 : UnitDelay  InitialCondition=eye(3)  SampleTime=-1  HasFrameUpgradeWarning=on
  Unit Delay4 : UnitDelay  InitialCondition=[S_ub0_ic_fps, S_vb0_ic_fps, S_wb0_ic_fps]  SampleTime=-1  HasFrameUpgradeWarning=on
  Unit Delay5 : UnitDelay  InitialCondition=[S_pb0_ic_dps, S_qb0_ic_dps, S_rb0_ic_dps]  SampleTime=-1  HasFrameUpgradeWarning=on
  Unit Delay6 : UnitDelay  InitialCondition=S_betad0_ic_deg  SampleTime=-1  HasFrameUpgradeWarning=on
  Unit Delay7 : UnitDelay  InitialCondition=S_alphad0_ic_deg  SampleTime=-1  HasFrameUpgradeWarning=on
  Unit Delay8 : UnitDelay  InitialCondition=[S_ub0_ic_fps, S_vb0_ic_fps, S_wb0_ic_fps]  SampleTime=-1  HasFrameUpgradeWarning=on
  "Vb, omega_b" : Scope  NumInputPorts=6
  Ve Scope : Scope  NumInputPorts=6
  alphad_deg1 : Outport
  betad_deg1 : Outport  Port=2
  delvl_state_deg : Outport  Port=3
  delvr_state_deg : Outport  Port=4
  drud_state_deg : Outport  Port=5
  fprop_state_lbf : Outport  Port=6
  vnorth_state_fps : Outport  Port=7
  veast_state_fps : Outport  Port=8
  vup_state_fps : Outport  Port=9
  xnorth_state_ft : Outport  Port=10
  xeast_state_ft : Outport  Port=11
  xup_state_ft : Outport  Port=12
  phi_state_rad : Outport  Port=13
  theta_state_rad : Outport  Port=14
  psi_state_rad : Outport  Port=15
  R_NEDtoB : Outport  Port=16
  ub_state_fps : Outport  Port=17
  vb_state_fps : Outport  Port=18
  wb_state_fps : Outport  Port=19
  pb_state_rps : Outport  Port=20
  qb_state_rps : Outport  Port=21
  rb_state_rps : Outport  Port=22
  pbdot_state_rps2 : Outport  Port=23
  qbdot_state_rps2 : Outport  Port=24
  rbdot_state_rps2 : Outport  Port=25
  axb_state_fps2 : Outport  Port=26
  ayb_state_fps2 : Outport  Port=27
  azb_state_fps2 : Outport  Port=28
  mach_state_nd : Outport  Port=29
  wires:
  Demux9/2 -> Ve Scope/2  "Vey"
  Demux7/1 -> "Vb, omega_b"/1  "Vbx"
  Demux8/2 -> "Vb, omega_b"/5  "q"
  Subsystem1/2(betad_deg) -> [betad_deg], betad_deg1/1
  [Vb_fps] -> Subsystem1/1(In1)
  Demux7/3 -> "Vb, omega_b"/3  "Vbz"
  Get Forces Moments/4(D) -> Scope1/2  "drag"
  Demux7/2 -> "Vb, omega_b"/2  "Vby"
  Demux8/3 -> "Vb, omega_b"/6  "r"
  Get Forces Moments/1(F) -> 6DOF (Euler Angles)1/1, Scope/1
  Demux10/1 -> Ve Scope/4  "Xex"
  Get Forces Moments/2(M) -> 6DOF (Euler Angles)1/2
  Demux9/1 -> Ve Scope/1  "Vex"
  Demux9/3 -> Ve Scope/3  "Vez"
  Subsystem1/1(alphad_deg) -> [alphad_deg], alphad_deg1/1
  Demux8/1 -> "Vb, omega_b"/4  "p"
  Demux10/2 -> Ve Scope/5  "Xey"
  Demux10/3 -> Ve Scope/6  "Xez"
  Get Forces Moments/3(L) -> Scope1/1  "lift"
  [Omegab_dps] -> Unit Delay5/1
  [Vb_fps] -> Unit Delay4/1
  [betad_deg] -> Unit Delay6/1
  [alphad_deg] -> Unit Delay7/1
  drud_deg/1 -> Unit Delay2/1
  [Vb_fps] -> Unit Delay8/1
  Constant1/1 -> Get Forces Moments/11(F_prop), fprop_state_lbf/1
  Constant2/1 -> Mach Number/2
  Mach Number/1 -> mach_state_nd/1, Get Forces Moments/10(mach)
  Constant/1 -> Get Forces Moments/9(rho_sl_ft3)
  Demux/3 -> vup_state_fps/1
  Demux5/3 -> rbdot_state_rps2/1
  Demux1/2 -> xeast_state_ft/1
  Demux/2 -> veast_state_fps/1
  6DOF (Euler Angles)1/4 -> [DCM], R_NEDtoB/1
  6DOF (Euler Angles)1/7 -> Demux5/1
  6DOF (Euler Angles)1/3 -> Demux2/1, [Omegab_dps]
  6DOF (Euler Angles)1/2 -> Demux1/1, Demux10/1
  Demux2/3 -> psi_state_rad/1
  Demux1/1 -> xnorth_state_ft/1
  6DOF (Euler Angles)1/6 -> Demux8/1, Demux4/1
  Demux6/1 -> axb_state_fps2/1
  Demux/1 -> vnorth_state_fps/1
  Demux5/2 -> qbdot_state_rps2/1
  Demux5/1 -> pbdot_state_rps2/1
  Demux4/2 -> qb_state_rps/1
  Demux4/1 -> pb_state_rps/1
  Demux2/1 -> phi_state_rad/1
  Demux4/3 -> rb_state_rps/1
  6DOF (Euler Angles)1/8 -> Demux6/1
  Demux3/3 -> wb_state_fps/1
  Demux6/3 -> azb_state_fps2/1
  Demux2/2 -> theta_state_rad/1
  Demux6/2 -> ayb_state_fps2/1
  6DOF (Euler Angles)1/1 -> Demux9/1, Demux/1
  Demux3/1 -> ub_state_fps/1
  Demux1/3 -> xup_state_ft/1
  Demux3/2 -> vb_state_fps/1
  6DOF (Euler Angles)1/5 -> [Vb_fps], Demux7/1, Demux3/1
  [DCM] -> Unit Delay3/1
  Sum1/1 -> delvl_state_deg/1, Get Forces Moments/4(delvl_deg)
  Sum/1 -> delvr_state_deg/1, Get Forces Moments/5(delvr_deg)
  symelv_cmd_deg/1 -> Unit Delay/1
  Unit Delay/1 -> Sum/1, Sum1/1
  difelv_cmd_deg/1 -> Unit Delay1/1
  Unit Delay1/1 -> Sum/2, Sum1/2
  Unit Delay2/1 -> Get Forces Moments/6(drud_deg), drud_state_deg/1
  Unit Delay3/1 -> Get Forces Moments/1(DCM)
  Unit Delay4/1 -> Get Forces Moments/2(V_b_fps)
  Unit Delay5/1 -> Get Forces Moments/3(Omega_b_dps)
  Unit Delay6/1 -> Get Forces Moments/7(betad_deg)
  Unit Delay7/1 -> Get Forces Moments/8(alphad_deg)
  Unit Delay8/1 -> Mach Number/1

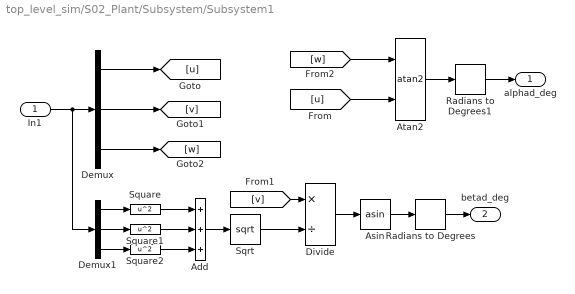
== system top_level_sim/S02_Plant/Subsystem/Subsystem1 ==
  In1 : Inport
  Add : Sum  Inputs=+++
  Asin : Trigonometry  Operator=asin
  Atan2 : Trigonometry  Operator=atan2
  Demux : Demux  Outputs=3
  Demux1 : Demux  Outputs=3
  Divide : Product  Inputs=*/
  Radians to Degrees : simulink_extras/Transformations/Radians to Degrees
  Radians to Degrees1 : simulink_extras/Transformations/Radians to Degrees
  Sqrt : Sqrt
  Square : Math  Operator=square
  Square1 : Math  Operator=square
  Square2 : Math  Operator=square
  alphad_deg : Outport
  betad_deg : Outport  Port=2
  wires:
  Atan2/1 -> Radians to Degrees1/1
  Asin/1 -> Radians to Degrees/1
  Divide/1 -> Asin/1
  Demux/3 -> [w]
  Demux/1 -> [u]
  Demux/2 -> [v]
  [w] -> Atan2/1
  [u] -> Atan2/2
  [v] -> Divide/1
  Radians to Degrees/1 -> betad_deg/1
  Radians to Degrees1/1 -> alphad_deg/1
  Sqrt/1 -> Divide/2
  Add/1 -> Sqrt/1
  In1/1 -> Demux1/1, Demux/1
  Demux1/1 -> Square/1
  Square1/1 -> Add/2
  Square/1 -> Add/1
  Demux1/2 -> Square1/1
  Demux1/3 -> Square2/1
  Square2/1 -> Add/3

== matlab function top_level_sim/CL04_NDIModule/Subsystem1/OnBoard Model ==
  data: rho_sl_ft3 input; DCM input; Xdot output single; Bmat output; alphad_deg input; betad_deg input; ub_fps input; vb_fps input; wb_fps input; mach input; pb_dps input; qb_dps input; rb_dps input; delvl_deg input; delvr_deg input; drud_deg input; fprop_lbf input; MASS_slg input; Ix_slgft2 input; Iy_slgft2 input; Iz_slgft2 input; Ixz_slgft2 input; Ixy_slgft2 input; Iyz_slgft2 input; Fgrav input; Bmat input double; n_col_calc input; Bcol_idx input int32; next_Bcol output; FM output
function [Xdot,Bmat,next_Bcol,FM] = fcn(rho_sl_ft3, DCM,alphad_deg, betad_deg,...
                              ub_fps,vb_fps,wb_fps,mach,...
                              pb_dps, qb_dps, rb_dps,...
                              delvl_deg, delvr_deg, drud_deg,fprop_lbf,...
                              MASS_slg, Ix_slgft2, Iy_slgft2, Iz_slgft2, Ixz_slgft2, Ixy_slgft2, Iyz_slgft2, ...
                              Fgrav, ...
                              Bmat, n_col_calc, Bcol_idx )
                          
    % Note: Only forces and moments are required output   
    % rho=0.00237;    % density, slug/ft^3
    % vtrue=0.0;      % true airspeed, ft/s
    % alt_agl=100.0;  % altitude AGL, ft
    % ub=0.1;        % body axis velocity, x, ft/s?
    % vb=0.0;        % body axis velocity, y, ft/s?
    % wb=0.0;        % body axis velocity, z, ft/s?
    % alphad=1.0;     % AoA of vehicle, deg
    % betad=0.0;      % AoS of vehicle, deg
    % delv_l_deg      % Left elevon deflection, deg; positive up
    % delv_r_deg      % Right elevon deflection, deg; positive up
    % drud_deg        % Rudder deflection, deg; positive left CHECK THIS
    % pb=0.0;         % body axis roll rate, deg/s; positive right wing down
    % qb=0.0;         % body axis pitch rate, deg/s; positive nose up
    % rb=0.0;         % body axis yaw rate, deg/s; positive nose right
    % REMOVED ROTOR RPMS BUT MIGHT NEED TO ADD IN SOMETHING FROM THE THRUST
    % MODEL
    % fscg=300.0;     % FSCG, inch; positive aft
    % blcg=0.0;       % BLCG, inch; positive to the right
    % wlcg=130.0;     % WLCG, inch; positive up


    

    % assert(isa(Fgrav,'single') && all(size(Fgrav)==[3,1]));
    % %Modify this assertion probably and the values below it
    % assert(isa(Bmat,'single') && all(size(Bmat)==[3,3]));
    % assert(isa(Bcol_idx,'int32') && all(size(Bcol_idx) == [1,1]));
    % assert(isa(n_col_calc,'int32') && all(size(n_col_calc) == [1,1]));
    % 
    D2R = single(pi/180);
    R2D = single(180/pi);
    
    V_b_fps = [ub_fps,vb_fps,wb_fps];
    Omega_b_dps = [pb_dps,qb_dps,rb_dps];
    %% Compute Xdot at the given flight condition
    % TESTING: alternatively, this result can be computed below by taking the average of the up & down perturbations
    [F, M, L, D] = getaeroforcesmoments(DCM,V_b_fps, Omega_b_dps, delvl_deg, delvr_deg, drud_deg, betad_deg, alphad_deg, rho_sl_ft3, mach, fprop_lbf);

    fnormb_lb = F(1);
    faxialb_lb = F(2);
    fsideb_lb = F(3);
    mpitchb_ftlb = M(1);
    lrollb_ftlb = M(2);
    nyawb_ftlb = M(3);

    Fx_b = faxialb_lb;
    Fy_b = fsideb_lb;
    Fz_b = fnormb_lb;  
    
    %WORK IN PROGRESS XDOT
    Xdot = state_derivs(  ub_fps, vb_fps, wb_fps, pb_dps*D2R, qb_dps*D2R, rb_dps*D2R, ...
                          Fx_b, Fy_b, Fz_b, lrollb_ftlb, mpitchb_ftlb, nyawb_ftlb, ...
                          MASS_slg, Ix_slgft2, Iy_slgft2, Iz_slgft2, Ixz_slgft2, Ixy_slgft2, Iyz_slgft2  );


	Xdot(4:6) = Xdot(4:6)*R2D;
    FM = [ Fx_b, Fy_b, Fz_b,  lrollb_ftlb, mpitchb_ftlb, nyawb_ftlb ];
    
% Removed for Load 2: BRG 6 Jul 2023
%     % These are used to store the average of the perturbation results to avoid an additional OBM call
%     Xdot_bar = single(zeros(6,1));
%     FM_bar = single(zeros(6,1));
    
%     %% Limit checking
%     % Limit the controls to just short of their max to ensure a B matrix column does not return as zero due to
%     % riding the limit
%     % FIXME: This needs to be made a little smarter than just limiting.
%     %       For example, we should prioritize diff_vane over sym_vane so we always have roll and yaw control.
%     %       Sym_vane is mainly used for acceleration. 
%     %       Similarly, differential collective should be prioritized over symmetric. By 'prioritize' I mean
%     %       the linear model should always be able to calculate the B matrix without riding the limits which
%     %       would lead to B matrix entries with zero effect.
%     vane_lim_OBM = single( 9.0 );
%     col_min_OBM = single( 7.0 );
%     col_max_OBM = single( 40. );
%     cyc_lim_OBM = single( 8.0 );
%     dvfl_deg = min(max(dvfl_deg,-vane_lim_OBM),vane_lim_OBM);
%     dvfr_deg = min(max(dvfr_deg,-vane_lim_OBM),vane_lim_OBM);
%     beta_plh_deg = min(max(beta_plh_deg,col_min_OBM),col_max_OBM);
%     beta_prh_deg = min(max(beta_prh_deg,col_min_OBM),col_max_OBM);
%     thet_1clh_deg = min(max(thet_1clh_deg,-cyc_lim_OBM),cyc_lim_OBM);
%     thet_1crh_deg = min(max(thet_1clh_deg,-cyc_lim_OBM),cyc_lim_OBM);
    

    %% Compute requested number of B matrix columns
    %NEED TO LOOK INTO THIS AND WHY THE SYM/DIF ARE FORMATTED THIS WAY
    U = single( [ 0.5*(delvl_deg + delvr_deg); % elevon_sym
                  0.5*(delvl_deg - delvr_deg); % elevon_dif
                  drud_deg]); % rudder
                

    nu = length(U);

    h = single(0.1); % controls perturbation size. For deflections in degrees, 0.2 is reasonable.  0.05 may be too small and produce undesired oscillation on table boundaries
    
    idx = [4,5,6]; % Select B-matrix columns.  (u,v,w,p,q,r = 1,2,3,4,5,6)
    nx = length(idx);
    
    assert(nu==3)
    assert(nx==3)
    

    

    icol = int32(min(max(1,Bcol_idx),nu)); % this is the first column to update
    %NEED TO UNDERSTAND HOW THE N_COL_CALC GETS UPDATED-its set to constant
    n_col_calc = int32(min(max(1,n_col_calc),nu)); % this is the number of columns to update starting from icol
    
    for in = 1:n_col_calc       
        
        Us = U(icol); % save orig control input
        
        % perturb dn
        U(icol) = Us-h;
        t_delvl_deg = U(1)+U(2);
        t_delvr_deg = U(1)-U(2);
        t_drud_deg = U(3);

        [F, M, L, D] = getaeroforcesmoments(DCM,V_b_fps, Omega_b_dps, t_delvl_deg, t_delvr_deg, t_drud_deg, betad_deg, alphad_deg, rho_sl_ft3, mach, 0);

        fnormb_lb = F(1);
        faxialb_lb = F(2);
        fsideb_lb = F(3);
        mpitchb_ftlb = M(1);
        lrollb_ftlb = M(2);
        nyawb_ftlb = M(3);

        Fx_b = faxialb_lb;
        Fy_b = fsideb_lb;
        Fz_b =  fnormb_lb;
        
% Removed for Load 2: BRG 6 Jul 2023        
%         FM_0 = [Fx_b; Fy_b; Fz_b; lrollb_ftlb; mpitchb_ftlb; nyawb_ftlb]; % for averaging forces/moments
                                     
        Xdot0 = state_derivs(  ub_fps, vb_fps, wb_fps, pb_dps*D2R, qb_dps*D2R, rb_dps*D2R, ...
                               Fx_b, Fy_b, Fz_b, lrollb_ftlb, mpitchb_ftlb, nyawb_ftlb, ...
                               MASS_slg, Ix_slgft2, Iy_slgft2, Iz_slgft2, Ixz_slgft2, Ixy_slgft2, Iyz_slgft2  );
        
        % perturb up
        U(icol) = Us+h;
        t_delvl_deg = U(1)+U(2);
        t_delvr_deg = U(1)-U(2);
        t_drud_deg = U(3);

        [F, M, L, D] = getaeroforcesmoments(DCM,V_b_fps, Omega_b_dps, t_delvl_deg, t_delvr_deg, t_drud_deg, betad_deg, alphad_deg, rho_sl_ft3, mach, 0);

        fnormb_lb = F(1);
        faxialb_lb = F(2);
        fsideb_lb = F(3);
        mpitchb_ftlb = M(1);
        lrollb_ftlb = M(2);
        nyawb_ftlb = M(3);
                                       
        Fx_b = faxialb_lb;
        Fy_b = fsideb_lb;
        Fz_b = fnormb_lb;
  
% Removed for Load 2: BRG 6 Jul 2023
%         FM_1 = [Fx_b; Fy_b; Fz_b; lrollb_ftlb; mpitchb_ftlb; nyawb_ftlb]; % for averaging forces/moments
                                     
        Xdot1 = state_derivs(  ub_fps, vb_fps, wb_fps, pb_dps*D2R, qb_dps*D2R, rb_dps*D2R, ...
                               Fx_b, Fy_b, Fz_b, lrollb_ftlb, mpitchb_ftlb, nyawb_ftlb, ...
                               MASS_slg, Ix_slgft2, Iy_slgft2, Iz_slgft2, Ixz_slgft2, Ixy_slgft2, Iyz_slgft2  );
        
        U(icol) = Us; % reset to original input
        
        % angular velocity output in deg/sec
        Xdot0(4:6) = Xdot0(4:6)*R2D;
        Xdot1(4:6) = Xdot1(4:6)*R2D;
      
% Removed for Load 2: BRG 6 Jul 2023
%         % Compute average Xdot_bar and FM_bar
%         if in==1
%             Xdot_bar = 0.5*(Xdot0 + Xdot1);
%             FM_bar = 0.5*(FM_0 + FM_1);
%         else
%             Xdot_bar = 0.5*( 0.5*(Xdot0 + Xdot1) + Xdot_bar );
%             FM_bar = 0.5*( 0.5*(FM_0+FM_1) + FM_bar );
%         end
        
        % Update Bmatrix
        Bmat(:,icol) = (Xdot1(idx)-Xdot0(idx))/(2*h); % update column icol
        
        % Update column index 
        icol =  icol + int32(1);
        if icol>nu
            icol = int32(1);
        end
    end
    
    
%     xdot_err = Xdot_bar-Xdot;
%     assert(all(abs(xdot_err) < 1e-2),'Xdot failed %10.5f, %10.5f, %10.5f, %10.5f, %10.5f,',xdot_err(1),xdot_err(2),xdot_err(3),xdot_err(4),xdot_err(5),xdot_err(6));
%     assert(all(abs(FM_bar-FM) < 1e-2),'FM failed');
    
    next_Bcol = icol;

end


%% THIS NEEDS TO BE CHECKED
function Xdot = state_derivs(u,v,w,p,q,r,Fx,Fy,Fz,Mx,My,Mz,MASS,Ix,Iy,Iz,Ixz,Ixy,Iyz)
    % Rigid Body Equations of Motion, linear and angular accel only
    %
    % Units are flexible but must be consistent, i.e.:
    %      [ft/s, lbs, ft-lbs, slugs, slug-ft^2]   or   [m/s, N, N-m, kg, kg-m^2]
    %                        (angular velocity in rad/sec always)
    %
    % Inputs:
    %    u,v,w: body axis velocity (x,y,z axes) in velocity units
    %    p,q,r: body axis angular velocity (x,y,z axes) in rad/sec
    %    Fx,Fy,Fz: body axis force (x,y,z axes) in force units. FORCE DUE TO GRAVITY SHALL BE INCLUDED.
    %    Mx,My,Mz: body axis moment (x,y,z axes) in moment units
    %    MASS: mass of the vehicle in mass units
    %
    %     Body axis coordinates:
    %         x: + forward
    %         y: + to the right
    %         z: + positive down
    %
    %    Ix,Iy,Iz,Ixz,Ixy,Iyz: moments of inertia in inertia units 
    %         Products of Inertia sign convention
    %         The sign convention used follows Stevens book & Durham's book:
    %              Ib = [[ Ixx, -Ixy, -Ixz],
    %                    [-Ixy,  Iyy, -Iyz],
    %                    [-Ixz, -Iyz, -Izz]]
    %              The products are defined as:  Ixy = sum(dm*x*y)
    %
    % Outputs:
    %    Xdot = [6x1] vector of [x,y,z] linear accels and [x,y,z] angular accels in body axes
    %
    coder.inline('always');
    
    
    Xdot=single(zeros(6,1));

    Xdot(1) = Fx/MASS - q*w + r*v;
    Xdot(2) = Fy/MASS - r*u + p*w;
    Xdot(3) = Fz/MASS - p*v + q*u;
    
    % TODO: handle angular momentum
    hx=0;
    hy=0;
    hz=0;

    % Angular Rate Derivatives
    % This is the expanded solution to w_dot_b = Ib^-1 * (Mb - OMGb*Ib*wb) for
    % the full inertia matrix
    %    Eq 2.8 Durham, Aircraft Control Allocation
    %    Eq 1.7-5 Stevens 2016, pg 37 - Note that Stevens inverse inertia matrix (1.7-6) is incorrect as of the 3rd edition
    Ixy = -Ixy; % follow negative convention
    Ixz = -Ixz; % follow negative convention
    Iyz = -Iyz; % follow negative convention
    idetI = 1.0/(Iy*(Ix*Iz-Ixz*Ixz) - Ix*Iyz*Iyz - Iz*Ixy*Ixy  + 2*Ixy*Ixz*Iyz); % reciprocal determinant of inertia matrix

    % intermediate results for  (Mb - OMGb*Ib*wb)
    t_Lres = Mx - q*( Iz*r+Iyz*q+Ixz*p + hz) + r*(Iyz*r+ Iy*q+Ixy*p + hy);
    t_Mres = My + p*( Iz*r+Iyz*q+Ixz*p + hz) - r*(Ixz*r+Ixy*q+ Ix*p + hx);
    t_Nres = Mz - p*(Iyz*r+ Iy*q+Ixy*p + hy) + q*(Ixz*r+Ixy*q+ Ix*p + hx);
    % p_dot
    Xdot(4) = idetI * (  (Iy*Iz - Iyz*Iyz) * t_Lres ...
                       + (Ixz*Iyz-Ixy*Iz)  * t_Mres ...
                       + (Ixy*Iyz-Ixz*Iy)  * t_Nres );
    % q_dot
    Xdot(5) = idetI * (  (Ixz*Iyz-Ixy*Iz)  * t_Lres ...
                       + (Ix*Iz - Ixz*Ixz) * t_Mres ...
                       + (Ixy*Ixz-Ix*Iyz)  * t_Nres );

    % r_dot
    Xdot(6) = idetI * (  (Ixy*Iyz-Ixz*Iy)  * t_Lres ...
                       + (Ixy*Ixz-Ix*Iyz)  * t_Mres ...
                       + (Ix*Iy - Ixy*Ixy) * t_Nres );
end

== matlab function top_level_sim/CL02_InputProcessing/Subsystem/MATLAB Function ==
  data: phi input; R_NEDtoB output; the input; psi input; R_NEtoGnd output
function [R_NEDtoB,R_NEtoGnd] = fcn(phi,the,psi)
% Compute two useful rotation matrices:
% input: 
%    phi: float, roll angle (rad)
%    the: float, pitch angle (rad)
%    psi: float, yaw angle (rad)
% output: 
%    Rib: [3x3] float, rotation from North-East-Down (NED) to body coordinates
%    Rig: [2x2] float, rotation from North-East ground plane speed to
%                      components aligned to longitudinal and lateral body 
%                      axes projected onto ground plane

    cphi = cos(phi);
    sphi = sin(phi);
    cthe = cos(the);
    sthe = sin(the);
    cpsi = cos(psi);
    spsi = sin(psi);
    
    % Rotation from NED to body:
    %      v_body = Rib * v_ned
    R_NEDtoB = [ cthe*cpsi                 cthe*spsi                -sthe      ;...
                 sphi*sthe*cpsi-cphi*spsi  sphi*sthe*spsi+cphi*cpsi  sphi*cthe ;...
                 cphi*sthe*cpsi+sphi*spsi  cphi*sthe*spsi-sphi*cpsi  cphi*cthe ];
        
    % Rotation from North&East ground speed to components aligned to 
    % projections of body x&y axes onto ground plane:  
    %      [Vgnd_xb;Vgnd_yb] = Rig * [Vnorth;Veast]
    R_NEtoGnd = [ cpsi     spsi;
                 -spsi    cpsi ];

end

== matlab function top_level_sim/S02_Plant/Subsystem/Get Forces Moments ==
  data: DCM input; V_b_fps input; Omega_b_dps input; delvl_deg input; F output; M output; delvr_deg input; drud_deg input; betad_deg input; alphad_deg input; rho_sl_ft3 input; mach input; F_prop input; L output; D output
function [F, M, L, D] = fcn(DCM,V_b_fps, Omega_b_dps, delvl_deg, delvr_deg, drud_deg, betad_deg, alphad_deg, rho_sl_ft3, mach, F_prop)
drud_deg
[F,M,L,D] = getaeroforcesmoments(DCM,V_b_fps, Omega_b_dps, delvl_deg, delvr_deg, drud_deg, betad_deg, alphad_deg, rho_sl_ft3, mach, F_prop);
